simulink model "shortcircuit"  (R2021a)
settings: Solver=ode45  StartTime=0.0  StopTime=10.0  RelTol=1e-3  EnableMultiTasking=on
libraries: spsRMSLib x10, spsCurrentMeasurementLib x4, spsVoltageMeasurementLib x4, spsMultiWindingTransformerLib x3, spsControlledVoltageSourceLib x3, spsPower3phInstantaneousLib x1, simulink x1, spspowerguiLib x1, spsGroundLib x1
settings Model: Creator=obulreddy  LastModifiedBy=mansi
settings SolverCC: AlgebraicLoopSolver=TrustRegion
settings DataIOCC: LimitDataPoints=on  SaveFormat=Array  ReturnWorkspaceOutputs=off
settings OptimizationCC: LifeSpan=inf
settings DebuggingCC: SFUnexpectedBacktrackingDiag=warning  SFNoUnconditionalDefaultTransitionDiag=warning  SFMachineParentedDataDiag=warning  ArithmeticOperatorsInVariantConditions=warning
settings HardwareCC: ProdBitPerPointer=32  ProdBitPerSizeT=32  ProdBitPerPtrDiffT=32  ProdLargestAtomicFloat=None  ProdIntDivRoundTo=Undefined  ProdEndianess=Unspecified  ProdWordSize=32  ProdHWDeviceType=32-bit Generic
settings ModelReferenceCC: PropagateSignalLabelsOutOfModel=off
settings SFSimCC: SimUseLocalCustomCode=off  CustomCodeUndefinedFunction=UseInterfaceOnly
settings RTWCC: RTWUseLocalCustomCode=off
settings CodeAppCC: StateflowObjectComments=on
settings GRTTargetCC: TargetLangStandard=C89/C90 (ANSI)
settings ConfigComp: CovMetricSettings=dw  CovSaveCumulativeToWorkspaceVar=on  CovSaveSingleToWorkspaceVar=on  CovExternalEMLEnable=off
settings SimscapeCC: SimscapeNormalizeSystem=off

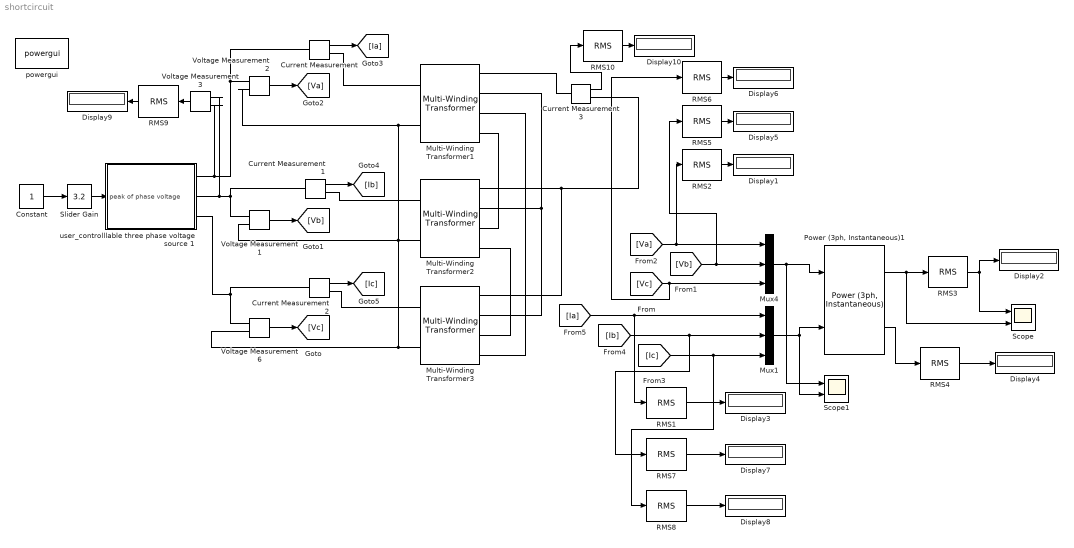
== system shortcircuit ==
  "Constant " : Constant
  Current Measurement{,1..3} (4 alike) : spsCurrentMeasurementLib/Current Measurement  PhasorSimulation=off  OutputType=Complex  PSBequivalent=0
  Display{1..10} (10 alike) : Display
  Multi-Winding Transformer1 : spsMultiWindingTransformerLib/Multi-Winding Transformer  LeftWindings=1  RightWindings=2  TappedWindings=no taps  NumberOfTaps=2  SetSaturation=off  Hysteresis=off  DataFile='hysteresis.mat'  Measurements=None  UNITS=SI  NominalPower=[2e3 50]  NominalVoltages="[ 133  66  115 ]"  WindingResistances=[0.040222 0.00689 0.029063]  WindingInductances=[0.00052306 0.00009866 0.00038096]  Rm=392.23  Lm=1.0076  Saturation=[0 0;0.051039 0.71845;21.266 0.91004]  BreakLoop=off  DiscreteSolver=Trapezoidal iterative  DataType=on  InitialFlux=0  TransfoNumber=1
      settings: SourceProductBaseCode=PS
  Multi-Winding Transformer2 : spsMultiWindingTransformerLib/Multi-Winding Transformer  LeftWindings=1  RightWindings=2  TappedWindings=no taps  NumberOfTaps=2  SetSaturation=off  Hysteresis=off  DataFile='hysteresis.mat'  Measurements=None  UNITS=SI  NominalPower=[2e3 50]  NominalVoltages="[ 133  66  115 ]"  WindingResistances=[0.040222 0.00689 0.029063]  WindingInductances=[0.00052306 0.00009866 0.00038096]  Rm=392.23  Lm=1.0076  Saturation=[0 0;0.051039 0.71845;21.266 0.91004]  BreakLoop=off  DiscreteSolver=Trapezoidal iterative  DataType=on  InitialFlux=0  TransfoNumber=1
      settings: SourceProductBaseCode=PS
  Multi-Winding Transformer3 : spsMultiWindingTransformerLib/Multi-Winding Transformer  LeftWindings=1  RightWindings=2  TappedWindings=no taps  NumberOfTaps=2  SetSaturation=off  Hysteresis=off  DataFile='hysteresis.mat'  Measurements=None  UNITS=SI  NominalPower=[2e3 50]  NominalVoltages="[ 133  66  115 ]"  WindingResistances=[0.040222 0.00689 0.029063]  WindingInductances=[0.00052306 0.00009866 0.00038096]  Rm=392.23  Lm=1.0076  Saturation=[0 0;0.051039 0.71845;21.266 0.91004]  BreakLoop=off  DiscreteSolver=Trapezoidal iterative  DataType=on  InitialFlux=0  TransfoNumber=1
      settings: SourceProductBaseCode=PS
  Mux1 : Mux  Inputs=3
  Mux4 : Mux  Inputs=3
  "Power (3ph, Instantaneous)1" : spsPower3phInstantaneousLib/Power (3ph, Instantaneous)
  RMS{1..10} (10 alike) : spsRMSLib/RMS  TrueRMS=on  Freq=50  RMSInit=0  Ts=0
  Scope : Scope  NumInputPorts=2
  Scope1 : Scope  NumInputPorts=2
  Slider Gain : simulink/Math Operations/Slider Gain  gain=3.2  low=0  high=30
  Voltage Measurement{1..3,6} (4 alike) : spsVoltageMeasurementLib/Voltage Measurement  PhasorSimulation=off  OutputType=Complex  PSBequivalent=0
  powergui : spspowerguiLib/powergui  Priority=1  SimulationMode=Continuous  SampleTime=50e-6  frequency=60  Iterations=50  frequencyindice=0  Pbase=100e6  ErrMax=1e-4  UnitsV=kV  UnitsW=MW  buscounter=0  FunctionMessages=off  echomessages=off  EnableUseOfTLC=off  CurrentSourceSwitches=off  DisableSnubberDevices=off  DisableRonSwitches=off  DisableVfSwitches=off  DisplayEquations=off  AutomaticDiscreteSolvers=off  SolverType=Tustin/Backward Euler (TBE)  Interpol=off  ExternalGateDelay=off  methode=off  Ts=100  x0status=blocks  SPID=on  SwTol=0  HookPort=off  NonlinearTolerance=1e-4  nMaxIteration=100  ContinueOnMaxIteration=off  RestoreLinks=warning  ResistiveCurrentMeasurement=off  Frange=[0:2:500]  Ylog=off  Xlog=on  ShowGrid=off  save=off  variable=ZData  structure=0  ZoomFFT=off  StartTime=0.0  cycles=1  DisplayStyle=1  fundamental=60  FreqAxis=off  MaxFrequency=1000  frequencyindicesteady=1  RmsSteady=1  display=off
  user_controlllable three phase voltage source 1 : Subsystem
  wires:
  [Ib] -> RMS7/1, Mux1/2
  RMS5/1 -> Display5/1
  Current Measurement1/1 -> [Ib]
  [Ic] -> RMS8/1, Mux1/3
  [Ia] -> Mux1/1, RMS1/1
  Current Measurement2/1 -> [Ic]
  RMS1/1 -> Display3/1
  RMS9/1 -> Display9/1
  Voltage Measurement6/1 -> [Vc]
  Current Measurement/1 -> [Ia]
  Voltage Measurement1/1 -> [Vb]
  "Power (3ph, Instantaneous)1"/2 -> RMS4/1
  [Vc] -> RMS6/1, Mux4/3
  "Power (3ph, Instantaneous)1"/1 -> Scope/2, RMS3/1
  RMS3/1 -> Display2/1, Scope/1
  Slider Gain/1 -> user_controlllable three phase voltage source 1/1(peak of phase voltage)
  RMS8/1 -> Display8/1
  RMS4/1 -> Display4/1
  Voltage Measurement3/1 -> RMS9/1
  RMS2/1 -> Display1/1
  Voltage Measurement2/1 -> [Va]
  RMS6/1 -> Display6/1
  Mux1/1 -> Scope1/2, "Power (3ph, Instantaneous)1"/2
  [Vb] -> RMS5/1, Mux4/2
  RMS7/1 -> Display7/1
  Mux4/1 -> Scope1/1, "Power (3ph, Instantaneous)1"/1
  "Constant "/1 -> Slider Gain/1
  [Va] -> RMS2/1, Mux4/1
  RMS10/1 -> Display10/1
  Current Measurement3/1 -> RMS10/1
  connections:
  Multi-Winding Transformer2/RConn2 -- Multi-Winding Transformer3/RConn2 -- Multi-Winding Transformer1/RConn2
  Current Measurement/LConn1 -- Voltage Measurement2/LConn1 -- Voltage Measurement3/LConn2 -- user_controlllable three phase voltage source 1/RConn1
  Voltage Measurement6/LConn1 -- user_controlllable three phase voltage source 1/RConn3 -- Current Measurement2/LConn1
  Current Measurement1/LConn1 -- Voltage Measurement1/LConn1 -- Voltage Measurement3/LConn1 -- user_controlllable three phase voltage source 1/RConn2
  Multi-Winding Transformer1/LConn2 -- Multi-Winding Transformer3/LConn2 -- Voltage Measurement6/LConn2 -- Voltage Measurement1/LConn2 -- Multi-Winding Transformer2/LConn2 -- Voltage Measurement2/LConn2
  Current Measurement/RConn1 -- Multi-Winding Transformer1/LConn1
  Current Measurement2/RConn1 -- Multi-Winding Transformer3/LConn1
  Multi-Winding Transformer3/RConn3 -- Multi-Winding Transformer2/RConn4
  Current Measurement1/RConn1 -- Multi-Winding Transformer2/LConn1
  Multi-Winding Transformer1/RConn4 -- Multi-Winding Transformer2/RConn3
  Multi-Winding Transformer3/RConn4 -- Multi-Winding Transformer1/RConn3
  Multi-Winding Transformer3/RConn1 -- Multi-Winding Transformer2/RConn1 -- Current Measurement3/RConn1
  Current Measurement3/LConn1 -- Multi-Winding Transformer1/RConn1

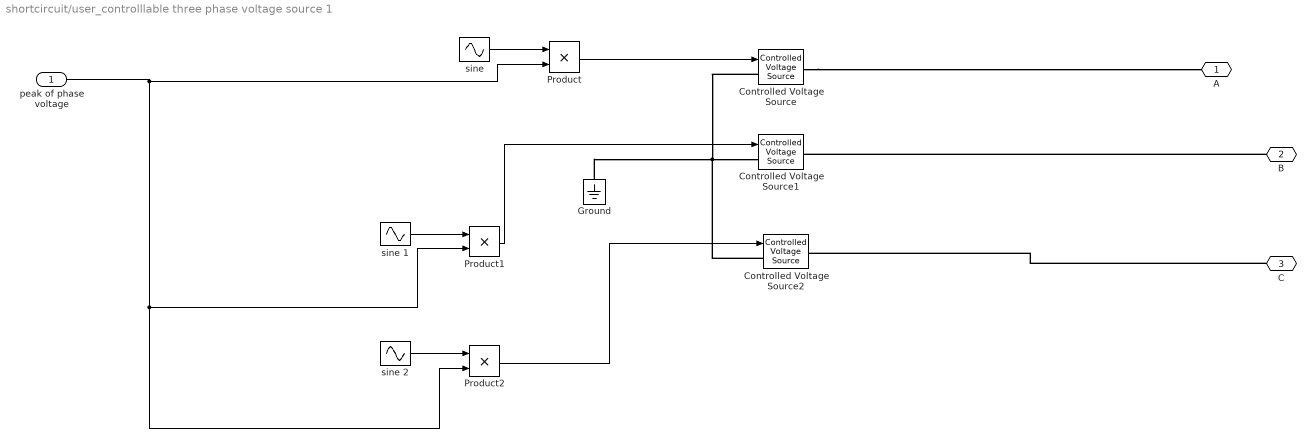
== system shortcircuit/user_controlllable three phase voltage source 1 ==
  peak of phase voltage : Inport
  Controlled Voltage Source : spsControlledVoltageSourceLib/Controlled Voltage Source  Initialize=off  Source_Type=DC  Amplitude=0  Phase=0  Frequency=50  Measurements=None
  Controlled Voltage Source1 : spsControlledVoltageSourceLib/Controlled Voltage Source  Initialize=off  Source_Type=DC  Amplitude=0  Phase=-120  Frequency=50  Measurements=None
  Controlled Voltage Source2 : spsControlledVoltageSourceLib/Controlled Voltage Source  Initialize=off  Source_Type=DC  Amplitude=0  Phase=120  Frequency=50  Measurements=None
  Ground : spsGroundLib/Ground  LConnTagsString=a
  Product : Product
  Product1 : Product
  Product2 : Product
  "sine " : Sin  Frequency=2*pi*50  SampleTime=0
  sine 1 : Sin  Frequency=2*pi*50  Phase=-2*pi/3  SampleTime=0
  sine 2 : Sin  Frequency=2*pi*50  Phase=+2*pi/3  SampleTime=0
  A : PMIOPort  Side=Right
  B : PMIOPort  Port=2  Side=Right
  C : PMIOPort  Port=3  Side=Right
  wires:
  Product/1 -> Controlled Voltage Source/1
  sine 2/1 -> Product2/1
  Product2/1 -> Controlled Voltage Source2/1
  "sine "/1 -> Product/1
  sine 1/1 -> Product1/1
  Product1/1 -> Controlled Voltage Source1/1
  peak of phase voltage/1 -> Product2/2, Product1/2, Product/2
  connections:
  Controlled Voltage Source/RConn1 -- A/RConn1
  Controlled Voltage Source/LConn1 -- Controlled Voltage Source2/LConn1 -- Ground/LConn1 -- Controlled Voltage Source1/LConn1
  B/RConn1 -- Controlled Voltage Source1/RConn1
  C/RConn1 -- Controlled Voltage Source2/RConn1
